simulink library "RCTblocks"  (R2022a)
settings: Solver=ode45  StartTime=0.0  StopTime=10.0  RelTol=1e-3
undefined symbols (not defined in the file or in its folder): sfun_multiplot, ureal
libraries: cstblocks x1
settings Model: FPTRunName=Active  Creator=The MathWorks, Inc.  LastModifiedBy=The MathWorks, Inc.
settings SolverCC: AlgebraicLoopSolver=TrustRegion
settings DataIOCC: LimitDataPoints=on  SaveFormat=Array  SignalLoggingSaveFormat=ModelDataLogs  ReturnWorkspaceOutputs=off
settings OptimizationCC: BlockReduction=off  BooleanDataType=off  ExpressionDepthLimit=2147483647  LifeSpan=inf
settings DebuggingCC: SaveWithParameterizedLinksMsg=none  UnderspecifiedInitializationDetection=Classic  MergeDetectMultiDrivingBlocksExec=none  SignalResolutionControl=TryResolveAllWithWarning  FcnCallInpInsideContextMsg=warning  UnconnectedInputMsg=warning  UnconnectedOutputMsg=warning  UnconnectedLineMsg=warning  StateNameClashWarn=warning  SymbolicDimsDataTypeCodeGenerationDiagnostic=none  SFUnexpectedBacktrackingDiag=warning  SFNoUnconditionalDefaultTransitionDiag=warning  SFExecutionAtInitializationDiag=none  SFMachineParentedDataDiag=warning  ArithmeticOperatorsInVariantConditions=warning
settings HardwareCC: ProdBitPerPointer=32  ProdBitPerSizeT=32  ProdBitPerPtrDiffT=32  ProdLargestAtomicFloat=None  ProdIntDivRoundTo=Undefined  ProdEndianess=Unspecified  ProdWordSize=32  ProdHWDeviceType=32-bit Generic  TargetUnknown=on
settings ModelReferenceCC: PropagateSignalLabelsOutOfModel=off
settings SFSimCC: SimUseLocalCustomCode=off  CustomCodeUndefinedFunction=UseInterfaceOnly
settings RTWCC: RTWUseLocalCustomCode=off  DLArmComputeVersion=19.05
settings CodeAppCC: StateflowObjectComments=on
settings GRTTargetCC: TargetLangStandard=C89/C90 (ANSI)  CombineOutputUpdateFcns=off  GRTInterface=on
settings ConfigComp: CovMetricSettings=dw  CovSaveCumulativeToWorkspaceVar=on  CovSaveSingleToWorkspaceVar=on  CovExternalEMLEnable=off

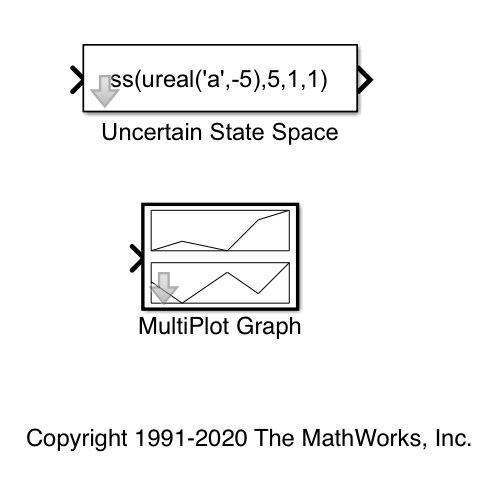
[thumbnail: Simulink's stored preview of the top-level diagram]
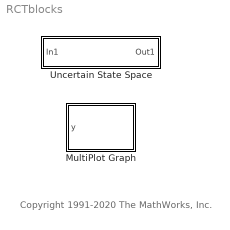
== system RCTblocks ==
  note: Copyright 1991-2020 The MathWorks, Inc.
  MultiPlot Graph : Subsystem  Tag=MultiPlot  LoadFcn=sfun_multiplot([],[],[],'LoadBlock')  StartFcn=sfun_multiplot([],[],[],'Start')  StopFcn=sfun_multiplot([],[],[],'Stop')  TreatAsAtomicUnit=on  SimViewingDevice=on  mask(MultiPlot Graph){tmin=0, tmax=20, ymin=-1, ymax=1, Tsamp=-1, titleString=, vnamesave=multisimout}
      mask prompts: tmin "Robust:simulink:maskPromptMultiPlotTMIN"; tmax "Robust:simulink:maskPromptMultiPlotTMAX"; ymin "Robust:simulink:maskPromptMultiPlotYMIN"; ymax "Robust:simulink:maskPromptMultiPlotYMAX"; Tsamp "Robust:simulink:maskPromptMultiPlotTS"; titleString "Robust:simulink:maskPromptMultiPlotTITLE"; vnamesave "Robust:simulink:maskPromptMultiPlotVAR"
      mask help: Robust:simulink:MultiPlotDesc
      mask init:
      | sfun_multiplot([],[],[],'MaskInitialize');
      settings: CopyFcn=sfun_multiplot([],[],[],'CopyBlock')  DeleteFcn=sfun_multiplot([],[],[],'DeleteBlock')  NameChangeFcn=sfun_multiplot([],[],[],'NameChange')
      mask Help: eval('rcthelp(''multiplot_graph'')')
      mask Callback tmin: sfun_multiplot([],[],[],'UpdateAxes')
      mask Callback tmax: sfun_multiplot([],[],[],'UpdateAxes')
      mask Callback ymin: sfun_multiplot([],[],[],'UpdateAxes')
      mask Callback ymax: sfun_multiplot([],[],[],'UpdateAxes')
      mask Callback titleString: sfun_multiplot([],[],[],'UpdateAxes')
      mask DialogControl tmin Prompt: t-min (view):
      mask DialogControl tmax Prompt: t-max (view):
      mask DialogControl ymin Prompt: y-min:
      mask DialogControl ymax Prompt: y-max:
      mask DialogControl Tsamp Prompt: Sample time:
      mask DialogControl titleString Prompt: Title:
      mask DialogControl vnamesave Prompt: Variable for Export to Workspace:
      mask Display:
      | plot([.05 .95 .95 .05 .05],[.05 .05 .45 .45 .05], [.05 .25 .55 .75 .95],[0.75 0.55 0.85 0.65 0.95]-0.5);
      | plot([.05 .95 .95 .05 .05],[.55 .55 .95 .95 .55], [.05 .25 .55 .75 .95],[0.55 0.65 0.55 0.85 0.95]);
  Uncertain State Space : Subsystem  Tag=USS  mask(Uncertain State Space Block){USystem=ss(ureal('a',-5),5,1,1), UValue=[], X0=[], uX0=[]}
      mask prompts: USystem "Robust:simulink:maskPromptUSS1"; UValue "Robust:simulink:maskPromptUSS2"; X0 "Robust:simulink:maskPromptUSS3"; uX0 "Robust:simulink:maskPromptUSS4"
      mask help: Robust:simulink:USSMaskDesc
      mask init:
      | try
      |    % read data to initialize mask variables
      |    [csys,cX0,sysname]=...
      |       USSMaskFcn('Initialize',gcb,USystem,UValue,X0,uX0);
      | catch ME
      |    csys = [];  cX0 = [];  sysname = '???';
      |    throw(ME)
      | end
      mask Help: eval('rcthelp(''uncertain_state_space_block'')')
      mask Callback USystem: USSMaskFcn('MaskUSSCallback',gcb);
      mask DialogControl USystem Prompt: Uncertain system variable (uss):
      mask DialogControl UValue Prompt: Uncertainty value (struct or [] to use nominal value):
      mask DialogControl X0 Prompt: Initial states (nominal dynamics):
      mask DialogControl uX0 Prompt: Initial states (uncertain dynamics):
      mask Display: disp(sysname)

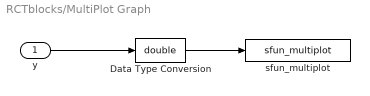
== system RCTblocks/MultiPlot Graph ==
  y : Inport
  Data Type Conversion : DataTypeConversion  OutDataTypeStr=double  SaturateOnIntegerOverflow=off  RndMeth=Floor
  sfun_multiplot : S-Function  FunctionName=sfun_multiplot  Parameters=tmin, tmax, ymin, ymax, Tsamp, titleString, vnamesave  SFunctionDeploymentMode=off  EnableBusSupport=off
  wires:
  y/1 -> Data Type Conversion/1
  Data Type Conversion/1 -> sfun_multiplot/1

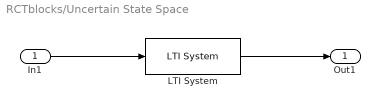
== system RCTblocks/Uncertain State Space ==
  In1 : Inport
  LTI System : cstblocks/LTI System  sys=csys  IC=cX0
  Out1 : Outport  VectorParamsAs1DForOutWhenUnconnected=off
  wires:
  In1/1 -> LTI System/1
  LTI System/1 -> Out1/1
